simulink model "g_s_cl2_old"  (Simulink 5.0)
settings: Solver=ode45  StartTime=t_init  StopTime=t_final  RelTol=1e-3
values from neighbouring files (symbols this model uses):
  C = [C Ck]    [polmul.m]
  D = D/D(1)    [tfvar.m]
  D1 = D    [tfvar.m]
undefined symbols (not defined in the file or in its folder): den, gamma, N1, num, R, S, st, st1, T, Ts
libraries: simulink x2
settings Model: Creator=kannan  LastModifiedBy=kannan  ExtModeAutoUpdateStatusClock=off

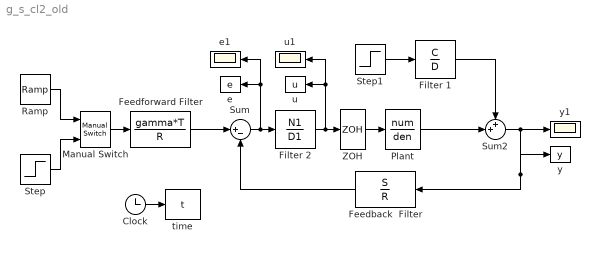
== system g_s_cl2_old ==
  " Filter 2" : DiscreteFilter  Numerator=N1  Denominator=D1  SampleTime=Ts
  Clock : Clock
      settings: Decimation=10
  Feedback  Filter : DiscreteFilter  Orientation=left  Numerator=S  Denominator=R  SampleTime=Ts
  Feedforward Filter : DiscreteFilter  Numerator=gamma*T  Denominator=R  SampleTime=Ts
  Filter 1 : DiscreteFilter  Numerator=C  Denominator=D  SampleTime=Ts
  Manual Switch : simulink/Signal Routing/Manual Switch  sw=0  action=0
  Plant : TransferFcn  Numerator=num  Denominator=den
  Ramp : simulink/Sources/Ramp  slope=1  start=0  X0=0
  Step : Step  Time=0  After=st  SampleTime=Ts
  Step1 : Step  Time=0  After=st1  SampleTime=Ts
  Sum : Sum  Inputs=|+-  SaturateOnIntegerOverflow=on
  Sum2 : Sum  Inputs=++|  SaturateOnIntegerOverflow=on
  ZOH : ZeroOrderHold  SampleTime=Ts
  e : ToWorkspace  VariableName=e  SampleTime=Ts  SaveFormat=Array
  e1 : Scope
      settings: YMin=-6e+164  YMax=1.02293e+149  SaveName=ScopeData2
  time : ToWorkspace  VariableName=t  SampleTime=Ts  SaveFormat=Array
  u : ToWorkspace  VariableName=u  SampleTime=Ts  SaveFormat=Array
  u1 : Scope
      settings: YMin=-6e+164  YMax=1.02293e+149
  y : ToWorkspace  VariableName=y  SampleTime=Ts  SaveFormat=Array
  y1 : Scope
      settings: YMin=-6e+164  YMax=1.02293e+149
  wires:
  Feedforward Filter/1 -> Sum/1
  Feedback  Filter/1 -> Sum/2
  Clock/1 -> time/1
  Plant/1 -> Sum2/2
  Filter 1/1 -> Sum2/1
  Step1/1 -> Filter 1/1
  Sum2/1 -> y1/1, Feedback  Filter/1, y/1
  Sum/1 -> " Filter 2"/1, e/1, e1/1
  " Filter 2"/1 -> u1/1, u/1, ZOH/1
  ZOH/1 -> Plant/1
  Ramp/1 -> Manual Switch/1
  Step/1 -> Manual Switch/2
  Manual Switch/1 -> Feedforward Filter/1
